simulink model "PMSM_Rs"  (R2024a)
settings: Solver=FixedStepDiscrete  StartTime=0.0  StopTime=0.5  FixedStep=1E-6  RelTol=1e-3
model workspace (MAT data in the model file):
  PWM_Frequency = Simulink.Parameter
  PWM_Frequency.Value = 30000
  PWM_Frequency.Complexity = 'real'
  PWM_Frequency.Dimensions = [1 1]
  PWM_Frequency.DataType = 'double'
  TimerPeriod = 0.1
values from neighbouring files (symbols this model uses):
  Flux = 0.01837    [Flux_Nonsensor_data_new.m]
undefined symbols (not defined in the file or in its folder): Down, Up
libraries: eePwmGenerator x11, slpidlib x3, spsDCVoltageSourceLib x2, spsPermanentMagnetSynchronousMachineLib x2, spsUniversalBridgeLib x2, sps_lib x1
settings Model: Creator=shish  LastModifiedBy=Administrator

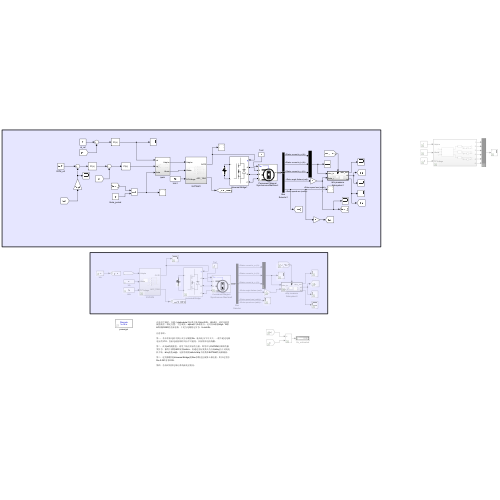
[thumbnail: Simulink's stored preview of the top-level diagram]
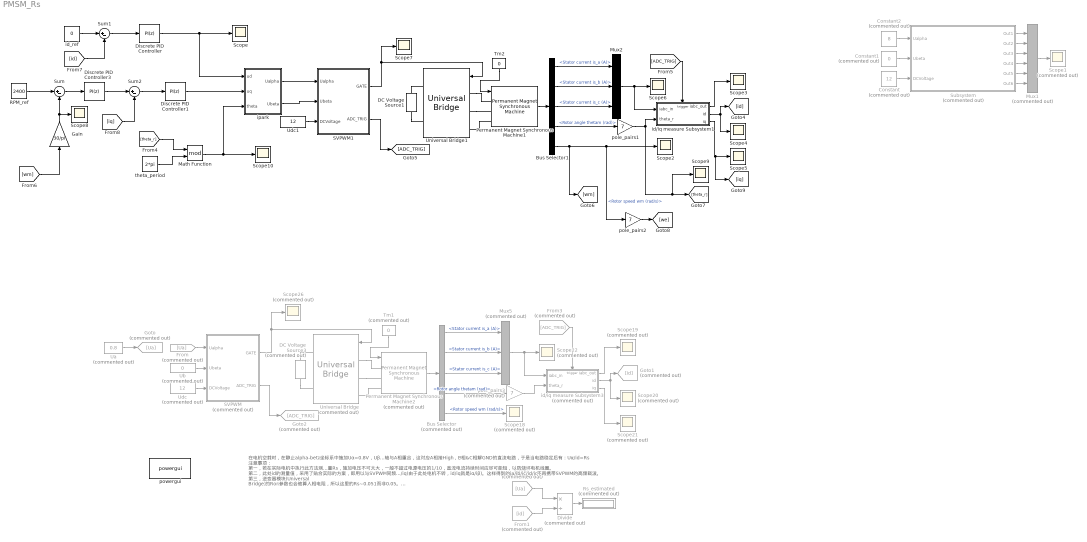
== system PMSM_Rs ==
  note: 在电机空载时，在静止alpha-beta坐标系中施加Uα=0.8V，Uβ=0V，此时电机将被强拖至一固定位置，不会旋转。alpha轴与A相重合，这对应A相接High，B相&C相解GND的直流电路，于是当电路稳定后有：Uα/id=Rs
      |
      | 注意事项：
      |
      | 第一，若在实际电机中执行此方法测量Rs，施加电压不可太大，一般不超过电源电压的1/10，直流电流持续时间应尽可能短，以防烧坏电机线圈。
      |
      | 第二，此处id的测量值，采用了贴合实际的方案，即用以与SVPWM同频率的触发信号，触发下桥臂ADC采样ia/ib/ic，再通过坐标变换人为合成id/iq(由于此处电机不转，id/iq就是iα/iβ)。这样得到的ia/ib/ic/id/iq不再携带SVPWM的高频载波。
      |
      | 第三，逆变器模块(Universal Bridge)的Ron参数也会被算入相电阻，所以这里的Rs~0.051而非0.05。
      |
      | 第四，仿真时间要足够让系统演化至稳态。
  Bus Selector : BusSelector  Commented=on  OutputSignals=Stator current is_a (A),Stator current is_b (A),Stator current is_c (A),Rotor angle thetam (rad),Rotor speed wm (rad/s)
  Bus Selector1 : BusSelector  OutputSignals=Stator current is_a (A),Stator current is_b (A),Stator current is_c (A),Rotor angle thetam (rad),Rotor speed wm (rad/s)
  Constant : Constant  Commented=on  Value=12
  Constant1 : Constant  Commented=on  Value=0
  Constant2 : Constant  Commented=on  Value=8
  DC Voltage Source1 : spsDCVoltageSourceLib/DC Voltage Source  Amplitude=12  Measurements=None
  DC Voltage Source3 : spsDCVoltageSourceLib/DC Voltage Source  Commented=on  Amplitude=12  Measurements=None
  Discrete PID Controller : slpidlib/PID Controller  Controller=PI  Form=Parallel  TimeDomain=Discrete-time  UseExternalTs=off  SampleTime=-1  IntegratorMethod=Forward Euler  FilterMethod=Forward Euler  ControllerParametersSource=internal  P=1000  I=5  UseKiTs=off  D=0  UseExternalDerivativeSource=off  N=100  UseFilter=on  TunerSelectOption=Transfer Function Based (PID Tuner App)  InitialConditionSource=internal  InitialConditionForIntegrator=0  InitialConditionForFilter=0  DifferentiatorICPrevScaledInput=0  ExternalReset=none  TrackingMode=off  Kt=1  LimitOutput=off  SatLimitsSource=internal  UpperSaturationLimit=inf  LowerSaturationLimit=-inf  LinearizeAsGain=off  AntiWindupMode=none  Kb=1  LimitIntegrator=off  UpperIntegratorSaturationLimit=inf  LowerIntegratorSaturationLimit=-inf  POutMin=[]  POutMax=[]  IOutMin=[]  IOutMax=[]  DOutMin=[]  DOutMax=[]  NOutMin=[]  NOutMax=[]  SumOutMin=[]  SumOutMax=[]  SaturationOutMin=[]  SaturationOutMax=[]  PParamMin=[]  PParamMax=[]  IParamMin=[]  IParamMax=[]  DParamMin=[]  DParamMax=[]  NParamMin=[]  NParamMax=[]  KbParamMin=[]  KbParamMax=[]  KtParamMin=[]  KtParamMax=[]  KbOutMin=[]  KbOutMax=[]  KtOutMin=[]  KtOutMax=[]  IntegratorOutMin=[]  IntegratorOutMax=[]  FilterOutMin=[]  FilterOutMax=[]  SumI1OutMin=[]  SumI1OutMax=[]  SumI2OutMin=[]  SumI2OutMax=[]  SumI3OutMin=[]  SumI3OutMax=[]  SumI4OutMin=[]  SumI4OutMax=[]  SumDOutMin=[]  SumDOutMax=[]  DifferentiatorOutMin=[]  DifferentiatorOutMax=[]  FilterDiffOutCoefMin=[]  FilterDiffOutCoefMax=[]  ReciprocalOutMin=[]  ReciprocalOutMax=[]  SumDenOutMin=[]  SumDenOutMax=[]  SumNumOutMin=[]  SumNumOutMax=[]  DivideOutMin=[]  DivideOutMax=[]  UdiffTsProdOutMin=[]  UdiffTsProdOutMax=[]  NTsProdOutMin=[]  NTsProdOutMax=[]  UintegralTsProdOutMin=[]  UintegralTsProdOutMax=[]  UngainTsProdOutMin=[]  UngainTsProdOutMax=[]  ClampingZeroOutDataTypeStr=Inherit: Inherit via back propagation  ClampingZeroOutMin=[]  ClampingZeroOutMax=[]  FilterDenConstantOutDataTypeStr=Inherit: Inherit via back propagation  FilterDenConstantOutMin=[]  FilterDenConstantOutMax=[]  PCopyOutDataTypeStr=Inherit: Inherit via back propagation  PCopyOutMin=[]  PCopyOutMax=[]  NCopyOutDataTypeStr=Inherit: Inherit via back propagation  NCopyOutMin=[]  NCopyOutMax=[]  IntegratorContinuousStateAttributes=''  IntegratorStateMustResolveToSignalObject=off  IntegratorRTWStateStorageClass=Auto  FilterContinuousStateAttributes=''  FilterStateMustResolveToSignalObject=off  FilterRTWStateStorageClass=Auto  ParallelPVariant=InternalParameters  IdealPVariant=Disabled  IVariant=InternalParameters  DVariant=Disabled  IntegratorVariant=Discrete  SatVariant=Disabled  AWVariant=Passthrough  PCopyVariant=Disabled  TRVariant=Disabled  FdbkBlocksVariant=Forward  IdealPFdbkVariant=Disabled  SatFdbkVariant=Disabled  DerivativeFilterVariant=Disabled  NVariant=Disabled  NCopyVariant=Disabled_SignalSpec  FilterICVariant=Disabled  IntegratorICVariant=InternalICs  ExternalResetVariant=Disabled  TRSumVariant=Passthrough  SumFdbkVariant=Disabled  SumVariant=Sum_PI  TsampFilterVariant=InternalTs  TsampNgainVariant=Passthrough  TsampIntegralVariant=Disabled_SignalSpec  ExternalSaturationOutDataTypeStr=Inherit: Same as second input  DerivativeSourceVariant=Disabled
      settings: LibrarySourceBlock=simulink/Discrete/Discrete PID Controller
  Discrete PID Controller1 : slpidlib/PID Controller  Controller=PI  Form=Parallel  TimeDomain=Discrete-time  UseExternalTs=off  SampleTime=-1  IntegratorMethod=Forward Euler  FilterMethod=Forward Euler  ControllerParametersSource=internal  P=1500  I=20  UseKiTs=off  D=0  UseExternalDerivativeSource=off  N=100  UseFilter=on  TunerSelectOption=Transfer Function Based (PID Tuner App)  InitialConditionSource=internal  InitialConditionForIntegrator=0  InitialConditionForFilter=0  DifferentiatorICPrevScaledInput=0  ExternalReset=none  TrackingMode=off  Kt=1  LimitOutput=off  SatLimitsSource=internal  UpperSaturationLimit=inf  LowerSaturationLimit=-inf  LinearizeAsGain=off  AntiWindupMode=none  Kb=1  LimitIntegrator=off  UpperIntegratorSaturationLimit=inf  LowerIntegratorSaturationLimit=-inf  POutMin=[]  POutMax=[]  IOutMin=[]  IOutMax=[]  DOutMin=[]  DOutMax=[]  NOutMin=[]  NOutMax=[]  SumOutMin=[]  SumOutMax=[]  SaturationOutMin=[]  SaturationOutMax=[]  PParamMin=[]  PParamMax=[]  IParamMin=[]  IParamMax=[]  DParamMin=[]  DParamMax=[]  NParamMin=[]  NParamMax=[]  KbParamMin=[]  KbParamMax=[]  KtParamMin=[]  KtParamMax=[]  KbOutMin=[]  KbOutMax=[]  KtOutMin=[]  KtOutMax=[]  IntegratorOutMin=[]  IntegratorOutMax=[]  FilterOutMin=[]  FilterOutMax=[]  SumI1OutMin=[]  SumI1OutMax=[]  SumI2OutMin=[]  SumI2OutMax=[]  SumI3OutMin=[]  SumI3OutMax=[]  SumI4OutMin=[]  SumI4OutMax=[]  SumDOutMin=[]  SumDOutMax=[]  DifferentiatorOutMin=[]  DifferentiatorOutMax=[]  FilterDiffOutCoefMin=[]  FilterDiffOutCoefMax=[]  ReciprocalOutMin=[]  ReciprocalOutMax=[]  SumDenOutMin=[]  SumDenOutMax=[]  SumNumOutMin=[]  SumNumOutMax=[]  DivideOutMin=[]  DivideOutMax=[]  UdiffTsProdOutMin=[]  UdiffTsProdOutMax=[]  NTsProdOutMin=[]  NTsProdOutMax=[]  UintegralTsProdOutMin=[]  UintegralTsProdOutMax=[]  UngainTsProdOutMin=[]  UngainTsProdOutMax=[]  ClampingZeroOutDataTypeStr=Inherit: Inherit via back propagation  ClampingZeroOutMin=[]  ClampingZeroOutMax=[]  FilterDenConstantOutDataTypeStr=Inherit: Inherit via back propagation  FilterDenConstantOutMin=[]  FilterDenConstantOutMax=[]  PCopyOutDataTypeStr=Inherit: Inherit via back propagation  PCopyOutMin=[]  PCopyOutMax=[]  NCopyOutDataTypeStr=Inherit: Inherit via back propagation  NCopyOutMin=[]  NCopyOutMax=[]  IntegratorContinuousStateAttributes=''  IntegratorStateMustResolveToSignalObject=off  IntegratorRTWStateStorageClass=Auto  FilterContinuousStateAttributes=''  FilterStateMustResolveToSignalObject=off  FilterRTWStateStorageClass=Auto  ParallelPVariant=InternalParameters  IdealPVariant=Disabled  IVariant=InternalParameters  DVariant=Disabled  IntegratorVariant=Discrete  SatVariant=Disabled  AWVariant=Passthrough  PCopyVariant=Disabled  TRVariant=Disabled  FdbkBlocksVariant=Forward  IdealPFdbkVariant=Disabled  SatFdbkVariant=Disabled  DerivativeFilterVariant=Disabled  NVariant=Disabled  NCopyVariant=Disabled_SignalSpec  FilterICVariant=Disabled  IntegratorICVariant=InternalICs  ExternalResetVariant=Disabled  TRSumVariant=Passthrough  SumFdbkVariant=Disabled  SumVariant=Sum_PI  TsampFilterVariant=InternalTs  TsampNgainVariant=Passthrough  TsampIntegralVariant=Disabled_SignalSpec  ExternalSaturationOutDataTypeStr=Inherit: Same as second input  DerivativeSourceVariant=Disabled
      settings: LibrarySourceBlock=simulink/Discrete/Discrete PID Controller
  Discrete PID Controller3 : slpidlib/PID Controller  Controller=PI  Form=Parallel  TimeDomain=Discrete-time  UseExternalTs=off  SampleTime=-1  IntegratorMethod=Forward Euler  FilterMethod=Forward Euler  ControllerParametersSource=internal  P=1500  I=10  UseKiTs=off  D=0  UseExternalDerivativeSource=off  N=100  UseFilter=on  TunerSelectOption=Transfer Function Based (PID Tuner App)  InitialConditionSource=internal  InitialConditionForIntegrator=0  InitialConditionForFilter=0  DifferentiatorICPrevScaledInput=0  ExternalReset=none  TrackingMode=off  Kt=1  LimitOutput=off  SatLimitsSource=internal  UpperSaturationLimit=inf  LowerSaturationLimit=-inf  LinearizeAsGain=off  AntiWindupMode=none  Kb=1  LimitIntegrator=off  UpperIntegratorSaturationLimit=inf  LowerIntegratorSaturationLimit=-inf  POutMin=[]  POutMax=[]  IOutMin=[]  IOutMax=[]  DOutMin=[]  DOutMax=[]  NOutMin=[]  NOutMax=[]  SumOutMin=[]  SumOutMax=[]  SaturationOutMin=[]  SaturationOutMax=[]  PParamMin=[]  PParamMax=[]  IParamMin=[]  IParamMax=[]  DParamMin=[]  DParamMax=[]  NParamMin=[]  NParamMax=[]  KbParamMin=[]  KbParamMax=[]  KtParamMin=[]  KtParamMax=[]  KbOutMin=[]  KbOutMax=[]  KtOutMin=[]  KtOutMax=[]  IntegratorOutMin=[]  IntegratorOutMax=[]  FilterOutMin=[]  FilterOutMax=[]  SumI1OutMin=[]  SumI1OutMax=[]  SumI2OutMin=[]  SumI2OutMax=[]  SumI3OutMin=[]  SumI3OutMax=[]  SumI4OutMin=[]  SumI4OutMax=[]  SumDOutMin=[]  SumDOutMax=[]  DifferentiatorOutMin=[]  DifferentiatorOutMax=[]  FilterDiffOutCoefMin=[]  FilterDiffOutCoefMax=[]  ReciprocalOutMin=[]  ReciprocalOutMax=[]  SumDenOutMin=[]  SumDenOutMax=[]  SumNumOutMin=[]  SumNumOutMax=[]  DivideOutMin=[]  DivideOutMax=[]  UdiffTsProdOutMin=[]  UdiffTsProdOutMax=[]  NTsProdOutMin=[]  NTsProdOutMax=[]  UintegralTsProdOutMin=[]  UintegralTsProdOutMax=[]  UngainTsProdOutMin=[]  UngainTsProdOutMax=[]  ClampingZeroOutDataTypeStr=Inherit: Inherit via back propagation  ClampingZeroOutMin=[]  ClampingZeroOutMax=[]  FilterDenConstantOutDataTypeStr=Inherit: Inherit via back propagation  FilterDenConstantOutMin=[]  FilterDenConstantOutMax=[]  PCopyOutDataTypeStr=Inherit: Inherit via back propagation  PCopyOutMin=[]  PCopyOutMax=[]  NCopyOutDataTypeStr=Inherit: Inherit via back propagation  NCopyOutMin=[]  NCopyOutMax=[]  IntegratorContinuousStateAttributes=''  IntegratorStateMustResolveToSignalObject=off  IntegratorRTWStateStorageClass=Auto  FilterContinuousStateAttributes=''  FilterStateMustResolveToSignalObject=off  FilterRTWStateStorageClass=Auto  ParallelPVariant=InternalParameters  IdealPVariant=Disabled  IVariant=InternalParameters  DVariant=Disabled  IntegratorVariant=Discrete  SatVariant=Disabled  AWVariant=Passthrough  PCopyVariant=Disabled  TRVariant=Disabled  FdbkBlocksVariant=Forward  IdealPFdbkVariant=Disabled  SatFdbkVariant=Disabled  DerivativeFilterVariant=Disabled  NVariant=Disabled  NCopyVariant=Disabled_SignalSpec  FilterICVariant=Disabled  IntegratorICVariant=InternalICs  ExternalResetVariant=Disabled  TRSumVariant=Passthrough  SumFdbkVariant=Disabled  SumVariant=Sum_PI  TsampFilterVariant=InternalTs  TsampNgainVariant=Passthrough  TsampIntegralVariant=Disabled_SignalSpec  ExternalSaturationOutDataTypeStr=Inherit: Same as second input  DerivativeSourceVariant=Disabled
      settings: LibrarySourceBlock=simulink/Discrete/Discrete PID Controller
  Divide : Product  Commented=on  Inputs=*/
  From : From  Commented=on  GotoTag=Ua
  From1 : From  Commented=on  GotoTag=id
  From2 : From  Commented=on  GotoTag=Ua
  From3 : From  Commented=on  GotoTag=ADC_TRIG
  Gain : Gain  Gain=30/pi
  Goto : Goto  Commented=on  GotoTag=Ua
  Goto1 : Goto  Commented=on  GotoTag=id
  Goto2 : Goto  Commented=on  GotoTag=ADC_TRIG
  Math Function : Math  Operator=mod
  Mux1 : Mux  Commented=on  Inputs=6
  Mux2 : Mux  Inputs=3
  Mux5 : Mux  Commented=on  Inputs=3
  Permanent Magnet Synchronous Machine1 : spsPermanentMagnetSynchronousMachineLib/Permanent Magnet Synchronous Machine  NbPhases=3  FluxDistribution=Sinusoidal  RotorType=Salient-pole  MechanicalLoad=Torque Tm  PresetModel=No  ShowDetailedParameters=on  MeasurementBus=off  Resistance=0.05  Inductance=8.5e-3  dqInductances=[1.8e-3,1.8e-3]  La=0.000395  MachineConstant=Flux linkage established by magnets (V.s)  Flux=0.00012  VoltageCst=0.15236  TorqueCst=0.00126  Flat=120  Mechanical=[0.000012 0.000005 7 0]  PolePairs=4  InitialConditions=[0,0, 0,0]  InitialConditions5ph=[0 0 0 0 0 0]  RefAngle=Aligned with phase A axis (original Park)  IterativeDiscreteModel=Trapezoidal non iterative  TsBlock=-1  TsPowergui=0
  Permanent Magnet Synchronous Machine2 : spsPermanentMagnetSynchronousMachineLib/Permanent Magnet Synchronous Machine  Commented=on  NbPhases=3  FluxDistribution=Sinusoidal  RotorType=Salient-pole  MechanicalLoad=Torque Tm  PresetModel=No  ShowDetailedParameters=on  MeasurementBus=off  Resistance=0.05  Inductance=8.5e-3  dqInductances=[1.8e-3,1.8e-3]  La=0.000395  MachineConstant=Flux linkage established by magnets (V.s)  Flux=0.00012  VoltageCst=0.15236  TorqueCst=0.00126  Flat=120  Mechanical=[0.000012 0.000005 7 0]  PolePairs=4  InitialConditions=[0,0, 0,0]  InitialConditions5ph=[0 0 0 0 0 0]  RefAngle=Aligned with phase A axis (original Park)  IterativeDiscreteModel=Trapezoidal non iterative  TsBlock=-1  TsPowergui=0
  RPM_ref : Constant  Value=2400
  Rs_estimated : Display  Commented=on
  SVPWM : Subsystem  Commented=on
  SVPWM1 : Subsystem
  Scope{,2..10} (10 alike) : Scope
  Scope{1,18..22,26} (7 alike) : Scope  Commented=on
  Subsystem : Subsystem  Commented=on
  Sum : Sum  Inputs=|+-
  Sum1 : Sum  Inputs=|+-
  Sum2 : Sum  Inputs=|+-
  Tm1 : Constant  Commented=on  Value=0
  Tm2 : Constant  Value=0
  Ua : Constant  Commented=on  Value=0.8
  Ub : Constant  Commented=on  Value=0
  Udc : Constant  Commented=on  Value=12
  Udc1 : Constant  Value=12
  Universal Bridge : spsUniversalBridgeLib/Universal Bridge  Commented=on  Arms=3  SnubberResistance=1e5  SnubberCapacitance=inf  Device=MOSFET / Diodes  Ron=1e-3  Lon=0  ForwardVoltages="[  0  0  ]"  ForwardVoltage=0  GTOparameters=[ 10e-6 , 20e-6 ]  IGBTparameters=[ 1e-6 , 2e-6 ]  Measurements=None  Measurements_2=None  converterType=Rectifier
  Universal Bridge1 : spsUniversalBridgeLib/Universal Bridge  Arms=3  SnubberResistance=1e5  SnubberCapacitance=inf  Device=MOSFET / Diodes  Ron=1e-3  Lon=0  ForwardVoltages="[  0  0  ]"  ForwardVoltage=0  GTOparameters=[ 10e-6 , 20e-6 ]  IGBTparameters=[ 1e-6 , 2e-6 ]  Measurements=None  Measurements_2=None  converterType=Rectifier
  id/iq measure Subsystem1 : Subsystem  TreatAsAtomicUnit=on
  id/iq measure Subsystem3 : Subsystem  Commented=on  TreatAsAtomicUnit=on
  id_ref : Constant  Value=0
  ipark : Subsystem
  pole_pairs1 : Gain  Gain=7
  pole_pairs2 : Gain  Gain=7
  pole_pairs3 : Gain  Commented=on  Gain=7
  powergui : sps_lib/powergui  Priority=1  SimulationMode=Discrete  SampleTime=1e-6  frequency=60  Iterations=50  frequencyindice=0  Pbase=100e6  ErrMax=1e-4  UnitsV=kV  UnitsW=MW  buscounter=0  FunctionMessages=off  echomessages=off  EnableUseOfTLC=off  CurrentSourceSwitches=off  DisableSnubberDevices=off  DisableRonSwitches=off  DisableVfSwitches=off  DisplayEquations=off  AutomaticDiscreteSolvers=off  SolverType=Tustin/Backward Euler (TBE)  Interpol=off  ExternalGateDelay=off  methode=off  Ts=100  x0status=blocks  SPID=on  SwTol=0  HookPort=off  NonlinearTolerance=1e-4  nMaxIteration=100  ContinueOnMaxIteration=off  RestoreLinks=warning  ResistiveCurrentMeasurement=off  Frange=[0:2:500]  Ylog=off  Xlog=on  ShowGrid=off  save=off  variable=ZData  structure=0  ZoomFFT=off  StartTime=0.0  cycles=1  DisplayStyle=1  fundamental=60  FreqAxis=off  MaxFrequency=1000  frequencyindicesteady=1  RmsSteady=1  display=off
  theta_period : Constant  Value=2*pi
  wires:
  Subsystem/1(Out1) -> Mux1/1
  Subsystem/2(Out2) -> Mux1/2
  Subsystem/3(Out3) -> Mux1/3
  Subsystem/4(Out4) -> Mux1/4
  Subsystem/5(Out5) -> Mux1/5
  Subsystem/6(Out6) -> Mux1/6
  Mux1/1 -> Scope1/1
  Constant/1 -> Subsystem/3(DCVoltage)
  Constant2/1 -> Subsystem/1(Ualpha)
  Constant1/1 -> Subsystem/2(Ubeta)
  Bus Selector/5 -> Scope18/1  "<Rotor speed wm (rad/s)>"
  Bus Selector/3 -> Mux5/3  "<Stator current is_c (A)>"
  Permanent Magnet Synchronous Machine2/1 -> Bus Selector/1
  Bus Selector/4 -> pole_pairs3/1  "<Rotor angle thetam (rad)>"
  Udc/1 -> SVPWM/3(DCVoltage)
  id/iq measure Subsystem3/1(iabc_out) -> Scope19/1
  Bus Selector/2 -> Mux5/2  "<Stator current is_b (A)>"
  Mux5/1 -> Scope22/1, id/iq measure Subsystem3/1(iabc_in)
  Tm1/1 -> Permanent Magnet Synchronous Machine2/1
  SVPWM/1(GATE) -> Universal Bridge/1, Scope26/1
  Bus Selector/1 -> Mux5/1  "<Stator current is_a (A)>"
  pole_pairs3/1 -> id/iq measure Subsystem3/2(theta_r)
  id/iq measure Subsystem3/2(id) -> Goto1/1, Scope20/1
  id/iq measure Subsystem3/3(iq) -> Scope21/1
  Ub/1 -> SVPWM/2(Ubeta)
  From/1 -> SVPWM/1(Ualpha)
  Ua/1 -> Goto/1
  From2/1 -> Divide/1
  From1/1 -> Divide/2
  Divide/1 -> Rs_estimated/1
  SVPWM/2(ADC_TRIG) -> Goto2/1
  From3/1 -> id/iq measure Subsystem3/Trigger
  [ADC_TRIG] -> id/iq measure Subsystem1/Trigger
  Tm2/1 -> Permanent Magnet Synchronous Machine1/1
  Bus Selector1/2 -> Mux2/2  "<Stator current is_b (A)>"
  Bus Selector1/1 -> Mux2/1  "<Stator current is_a (A)>"
  Bus Selector1/3 -> Mux2/3  "<Stator current is_c (A)>"
  id/iq measure Subsystem1/3(iq) -> [iq], Scope5/1
  SVPWM1/2(ADC_TRIG) -> [ADC_TRIG]
  id/iq measure Subsystem1/2(id) -> [id], Scope4/1
  Mux2/1 -> Scope6/1, id/iq measure Subsystem1/1(iabc_in)
  ipark/1(Ualpha) -> SVPWM1/1(Ualpha)
  id/iq measure Subsystem1/1(iabc_out) -> Scope3/1
  Permanent Magnet Synchronous Machine1/1 -> Bus Selector1/1
  Bus Selector1/5 -> pole_pairs2/1, Scope2/1, [wm]  "<Rotor speed wm (rad/s)>"
  Bus Selector1/4 -> pole_pairs1/1  "<Rotor angle thetam (rad)>"
  Udc1/1 -> SVPWM1/3(DCVoltage)
  pole_pairs1/1 -> Scope9/1, [theta_r], id/iq measure Subsystem1/2(theta_r)
  SVPWM1/1(GATE) -> Universal Bridge1/1, Scope7/1
  pole_pairs2/1 -> [we]
  [wm] -> Gain/1
  Sum/1 -> Discrete PID Controller3/1
  [id] -> Sum1/2
  Sum1/1 -> Discrete PID Controller/1
  [iq] -> Sum2/2
  id_ref/1 -> Sum1/1
  ipark/2(Ubeta) -> SVPWM1/2(Ubeta)
  Discrete PID Controller/1 -> ipark/1(ud), Scope/1
  Gain/1 -> Sum/2, Scope8/1
  RPM_ref/1 -> Sum/1
  Discrete PID Controller3/1 -> Sum2/1
  Sum2/1 -> Discrete PID Controller1/1
  Discrete PID Controller1/1 -> ipark/2(uq)
  [theta_r] -> Math Function/1
  theta_period/1 -> Math Function/2
  Math Function/1 -> Scope10/1, ipark/3(theta)
  connections:
  Universal Bridge/LConn2 -- Permanent Magnet Synchronous Machine2/LConn2
  Universal Bridge/LConn1 -- Permanent Magnet Synchronous Machine2/LConn1
  DC Voltage Source3/RConn1 -- Universal Bridge/RConn1
  Universal Bridge/LConn3 -- Permanent Magnet Synchronous Machine2/LConn3
  DC Voltage Source3/LConn1 -- Universal Bridge/RConn2
  DC Voltage Source1/LConn1 -- Universal Bridge1/RConn2
  Universal Bridge1/LConn1 -- Permanent Magnet Synchronous Machine1/LConn1
  Universal Bridge1/LConn3 -- Permanent Magnet Synchronous Machine1/LConn3
  DC Voltage Source1/RConn1 -- Universal Bridge1/RConn1
  Universal Bridge1/LConn2 -- Permanent Magnet Synchronous Machine1/LConn2

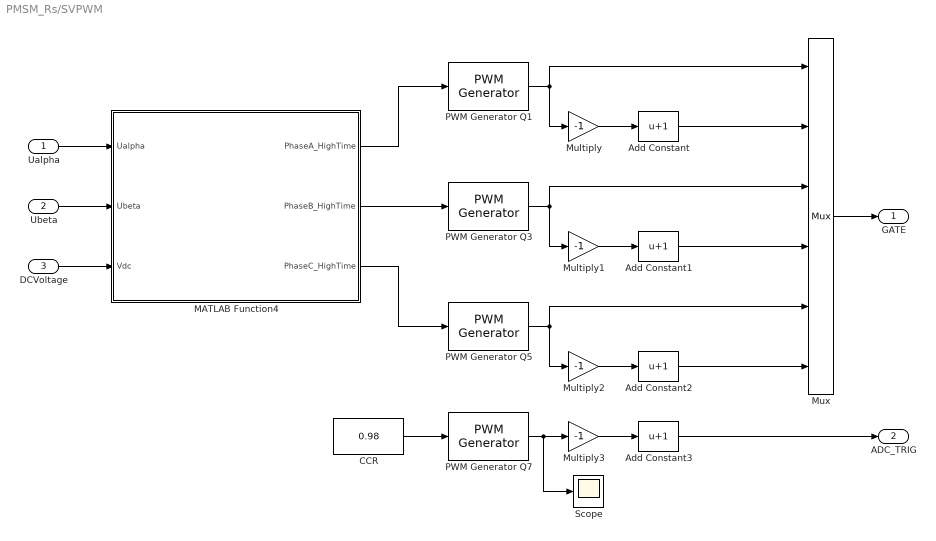
== system PMSM_Rs/SVPWM ==
  Ualpha : Inport
  Ubeta : Inport  Port=2
  DCVoltage : Inport  Port=3
  Add Constant{,1..3} (4 alike) : Bias  Bias=1  SaturateOnIntegerOverflow=off
  CCR : Constant  Value=0.98
  MATLAB Function4 : MATLAB Function  TreatAsAtomicUnit=on
  Multiply{,1..3} (4 alike) : Gain  Gain=-1
  Mux : Mux  Inputs=6
  PWM Generator Q{1,3,5,7} (4 alike) : eePwmGenerator/PWM Generator  CarrCount=Up-Down  Tper=1.0/PWM_Frequency  Tdelay=0  Ts=1E-6
  Scope : Scope
  GATE : Outport
  ADC_TRIG : Outport  Port=2
  wires:
  PWM Generator Q5/1 -> Mux/5, Multiply2/1
  PWM Generator Q1/1 -> Multiply/1, Mux/1
  Add Constant1/1 -> Mux/4
  Ubeta/1 -> MATLAB Function4/2(Ubeta)
  DCVoltage/1 -> MATLAB Function4/3(Vdc)
  MATLAB Function4/3(PhaseC_HighTime) -> PWM Generator Q5/1
  Multiply/1 -> Add Constant/1
  Multiply2/1 -> Add Constant2/1
  Add Constant/1 -> Mux/2
  MATLAB Function4/2(PhaseB_HighTime) -> PWM Generator Q3/1
  Add Constant2/1 -> Mux/6
  Multiply1/1 -> Add Constant1/1
  MATLAB Function4/1(PhaseA_HighTime) -> PWM Generator Q1/1
  Ualpha/1 -> MATLAB Function4/1(Ualpha)
  PWM Generator Q3/1 -> Mux/3, Multiply1/1
  PWM Generator Q7/1 -> Scope/1, Multiply3/1
  CCR/1 -> PWM Generator Q7/1
  Add Constant3/1 -> ADC_TRIG/1
  Multiply3/1 -> Add Constant3/1
  Mux/1 -> GATE/1

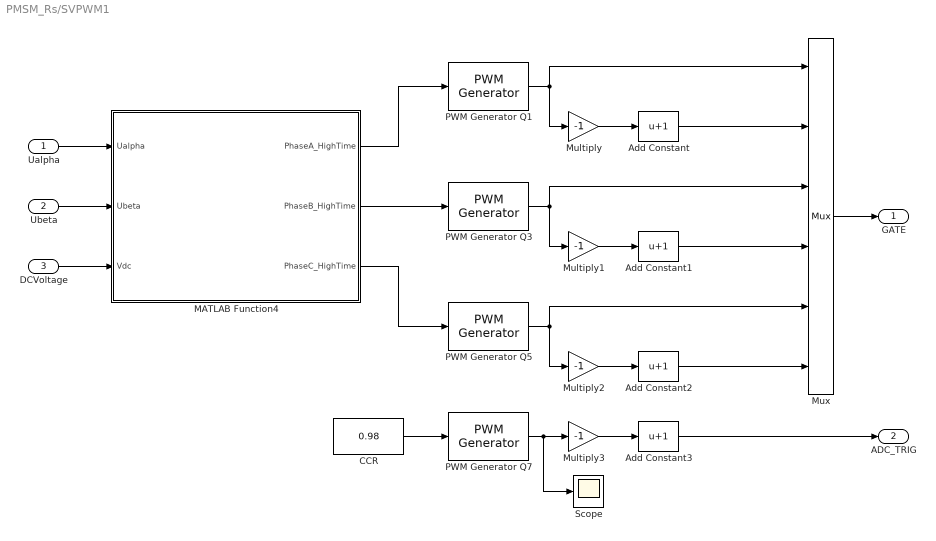
== system PMSM_Rs/SVPWM1 ==
  Ualpha : Inport
  Ubeta : Inport  Port=2
  DCVoltage : Inport  Port=3
  Add Constant{,1..3} (4 alike) : Bias  Bias=1  SaturateOnIntegerOverflow=off
  CCR : Constant  Value=0.98
  MATLAB Function4 : MATLAB Function  TreatAsAtomicUnit=on
  Multiply{,1..3} (4 alike) : Gain  Gain=-1
  Mux : Mux  Inputs=6
  PWM Generator Q{1,3,5,7} (4 alike) : eePwmGenerator/PWM Generator  CarrCount=Up-Down  Tper=1.0/PWM_Frequency  Tdelay=0  Ts=1E-6
  Scope : Scope
  GATE : Outport
  ADC_TRIG : Outport  Port=2
  wires:
  PWM Generator Q5/1 -> Mux/5, Multiply2/1
  PWM Generator Q1/1 -> Multiply/1, Mux/1
  Add Constant1/1 -> Mux/4
  Ubeta/1 -> MATLAB Function4/2(Ubeta)
  DCVoltage/1 -> MATLAB Function4/3(Vdc)
  MATLAB Function4/3(PhaseC_HighTime) -> PWM Generator Q5/1
  Multiply/1 -> Add Constant/1
  Multiply2/1 -> Add Constant2/1
  Add Constant/1 -> Mux/2
  MATLAB Function4/2(PhaseB_HighTime) -> PWM Generator Q3/1
  Add Constant2/1 -> Mux/6
  Multiply1/1 -> Add Constant1/1
  MATLAB Function4/1(PhaseA_HighTime) -> PWM Generator Q1/1
  Ualpha/1 -> MATLAB Function4/1(Ualpha)
  PWM Generator Q3/1 -> Mux/3, Multiply1/1
  PWM Generator Q7/1 -> Scope/1, Multiply3/1
  CCR/1 -> PWM Generator Q7/1
  Add Constant3/1 -> ADC_TRIG/1
  Multiply3/1 -> Add Constant3/1
  Mux/1 -> GATE/1

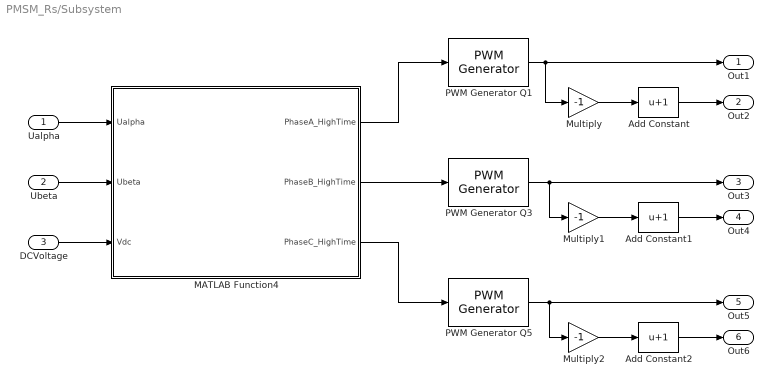
== system PMSM_Rs/Subsystem ==
  Ualpha : Inport
  Ubeta : Inport  Port=2
  DCVoltage : Inport  Port=3
  Add Constant : Bias  Bias=1  SaturateOnIntegerOverflow=off
  Add Constant1 : Bias  Bias=1  SaturateOnIntegerOverflow=off
  Add Constant2 : Bias  Bias=1  SaturateOnIntegerOverflow=off
  MATLAB Function4 : MATLAB Function  TreatAsAtomicUnit=on
  Multiply : Gain  Gain=-1
  Multiply1 : Gain  Gain=-1
  Multiply2 : Gain  Gain=-1
  PWM Generator Q1 : eePwmGenerator/PWM Generator  CarrCount=Up-Down  Tper=0.1  Tdelay=0  Ts=1E-5
  PWM Generator Q3 : eePwmGenerator/PWM Generator  CarrCount=Up-Down  Tper=0.1  Tdelay=0  Ts=1E-5
  PWM Generator Q5 : eePwmGenerator/PWM Generator  CarrCount=Up-Down  Tper=0.1  Tdelay=0  Ts=1E-5
  Out1 : Outport
  Out2 : Outport  Port=2
  Out3 : Outport  Port=3
  Out4 : Outport  Port=4
  Out5 : Outport  Port=5
  Out6 : Outport  Port=6
  wires:
  PWM Generator Q5/1 -> Out5/1, Multiply2/1
  PWM Generator Q1/1 -> Out1/1, Multiply/1
  Add Constant1/1 -> Out4/1
  Ubeta/1 -> MATLAB Function4/2(Ubeta)
  DCVoltage/1 -> MATLAB Function4/3(Vdc)
  MATLAB Function4/3(PhaseC_HighTime) -> PWM Generator Q5/1
  Multiply/1 -> Add Constant/1
  Multiply2/1 -> Add Constant2/1
  Add Constant/1 -> Out2/1
  MATLAB Function4/2(PhaseB_HighTime) -> PWM Generator Q3/1
  Add Constant2/1 -> Out6/1
  Multiply1/1 -> Add Constant1/1
  MATLAB Function4/1(PhaseA_HighTime) -> PWM Generator Q1/1
  Ualpha/1 -> MATLAB Function4/1(Ualpha)
  PWM Generator Q3/1 -> Out3/1, Multiply1/1

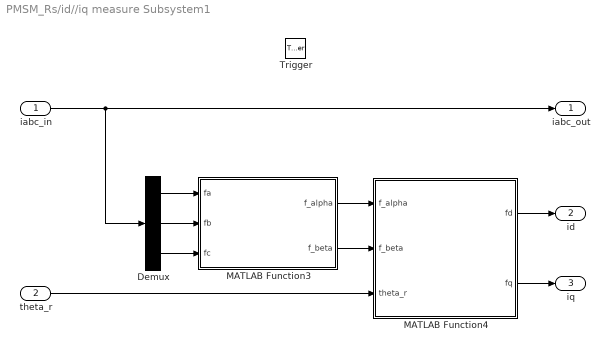
== system PMSM_Rs/id//iq measure Subsystem1 ==
  iabc_in : Inport
  theta_r : Inport  Port=2
  Trigger : TriggerPort  VariantControl=(inherit)
  Demux : Demux  Outputs=3
  MATLAB Function3 : MATLAB Function  TreatAsAtomicUnit=on
  MATLAB Function4 : MATLAB Function  TreatAsAtomicUnit=on
  iabc_out : Outport
  id : Outport  Port=2
  iq : Outport  Port=3
  wires:
  iabc_in/1 -> Demux/1, iabc_out/1
  Demux/3 -> MATLAB Function3/3(fc)
  Demux/2 -> MATLAB Function3/2(fb)
  Demux/1 -> MATLAB Function3/1(fa)
  MATLAB Function3/1(f_alpha) -> MATLAB Function4/1(f_alpha)
  MATLAB Function3/2(f_beta) -> MATLAB Function4/2(f_beta)
  theta_r/1 -> MATLAB Function4/3(theta_r)
  MATLAB Function4/1(fd) -> id/1
  MATLAB Function4/2(fq) -> iq/1

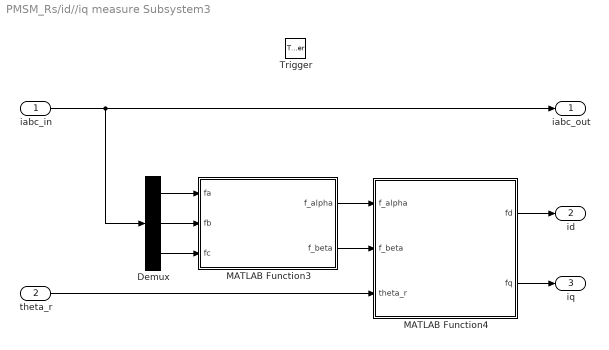
== system PMSM_Rs/id//iq measure Subsystem3 ==
  iabc_in : Inport
  theta_r : Inport  Port=2
  Trigger : TriggerPort  VariantControl=(inherit)
  Demux : Demux  Outputs=3
  MATLAB Function3 : MATLAB Function  TreatAsAtomicUnit=on
  MATLAB Function4 : MATLAB Function  TreatAsAtomicUnit=on
  iabc_out : Outport
  id : Outport  Port=2
  iq : Outport  Port=3
  wires:
  iabc_in/1 -> Demux/1, iabc_out/1
  Demux/3 -> MATLAB Function3/3(fc)
  Demux/2 -> MATLAB Function3/2(fb)
  Demux/1 -> MATLAB Function3/1(fa)
  MATLAB Function3/1(f_alpha) -> MATLAB Function4/1(f_alpha)
  MATLAB Function3/2(f_beta) -> MATLAB Function4/2(f_beta)
  theta_r/1 -> MATLAB Function4/3(theta_r)
  MATLAB Function4/1(fd) -> id/1
  MATLAB Function4/2(fq) -> iq/1

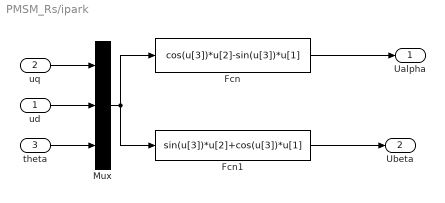
== system PMSM_Rs/ipark ==
  ud : Inport
  uq : Inport  Port=2
  theta : Inport  Port=3
  Fcn : Fcn  Expr=cos(u[3])*u[2]-sin(u[3])*u[1]
  Fcn1 : Fcn  Expr=sin(u[3])*u[2]+cos(u[3])*u[1]
  Mux : Mux  Inputs=3
  Ualpha : Outport
  Ubeta : Outport  Port=2
  wires:
  Mux/1 -> Fcn/1, Fcn1/1
  ud/1 -> Mux/2
  theta/1 -> Mux/3
  uq/1 -> Mux/1
  Fcn1/1 -> Ubeta/1
  Fcn/1 -> Ualpha/1

== matlab function PMSM_Rs/SVPWM1/MATLAB Function4 ==
  data: Ualpha input; PhaseA_HighTime output; Ubeta input; Vdc input; PhaseB_HighTime output; PhaseC_HighTime output
function [PhaseA_HighTime,PhaseB_HighTime,PhaseC_HighTime] = SVPWM_calculate(Ualpha,Ubeta,Vdc)

% unit:V %

%step 1,which sector?%
if Ualpha >= 0
    %sector=1,2,5,6%
    if Ubeta >= 0
        %sector=1,2%
        if Ubeta > sqrt(3)*Ualpha
            sector=2;
        else
            sector=1;
        end
    else
        %sector=5,6%
        if -Ubeta > sqrt(3)*Ualpha
            sector=5;
        else
            sector=6;
        end
    end
else
    %sector=2,3,4,5%
    if Ubeta >= 0
        %sector=2,3%
        if Ubeta > -sqrt(3)*Ualpha
            sector=2;
        else
            sector=3;
        end
    else
        %sector=4,5%
        if -Ubeta > -sqrt(3)*Ualpha
            sector=5;
        else
            sector=4;
        end
    end
end

%step 2,vector decompose%
v1 = (2*Vdc/3)*[ 1,0];
v2 = (2*Vdc/3)*[ 0.5, 0.5*sqrt(3)];
v3 = (2*Vdc/3)*[-0.5, 0.5*sqrt(3)];
v4 = (2*Vdc/3)*[-1,0];
v5 = (2*Vdc/3)*[-0.5,-0.5*sqrt(3)];
v6 = (2*Vdc/3)*[ 0.5,-0.5*sqrt(3)];

if sector == 1
    vm=v1;vn=v2;
elseif sector == 2
    vm=v2;vn=v3;
elseif sector == 3
    vm=v3;vn=v4;
elseif sector == 4
    vm=v4;vn=v5;
elseif sector == 5
    vm=v5;vn=v6;
else
    vm=v6;vn=v1;
end

cm = (Ualpha*vn(2) - Ubeta*vn(1))/(vm(1)*vn(2) - vm(2)*vn(1));

if abs(vn(1))>1e-7
    cn = (Ualpha-cm*vm(1))/vn(1);
else
    cn = (Ubeta-cm*vm(2))/vn(2);
end
c_summ = cm+cn;
% if c_summ > 1
%     cm = cm/c_summ;
%     cn = cn/c_summ;
% end
if c_summ > 0.95
    cm = 0.95*cm/c_summ;
    cn = 0.95*cn/c_summ;
end

c0 = (1-cm-cn);
c0 = 0.5*c0;
c7 = c0;

%step 3,duty cycle%
if sector == 1
    %v1:100  v2:110%
    PhaseA_HighTime = cm+cn+c7;
    PhaseB_HighTime = cn+c7;
    PhaseC_HighTime = c7;
elseif sector == 2
    %v2:110  v3:010%
    PhaseA_HighTime = cm+c7;
    PhaseB_HighTime = cm+cn+c7;
    PhaseC_HighTime = c7;
elseif sector == 3
    %v3:010  v4:011%
    PhaseA_HighTime = c7;
    PhaseB_HighTime = cm+cn+c7;
    PhaseC_HighTime = cn+c7;
elseif sector == 4
    %v4:011  v5:001%
    PhaseA_HighTime = c7;
    PhaseB_HighTime = cm+c7;
    PhaseC_HighTime = cm+cn+c7;
elseif sector == 5
    %v5:001  v6:101%
    PhaseA_HighTime = cn+c7;
    PhaseB_HighTime = c7;
    PhaseC_HighTime = cm+cn+c7;
else
    %v6:101  v1:100%
    PhaseA_HighTime = cm+cn+c7;
    PhaseB_HighTime = c7;
    PhaseC_HighTime = cm+c7;
end

== matlab function PMSM_Rs/id//iq measure Subsystem1/MATLAB Function3 ==
  data: fa input; f_alpha output; fb input; fc input; f_beta output
function [f_alpha,f_beta]= ABC_to_AlphaBeta(fa,fb,fc)
f_alpha = (2/3)*(fa-0.5*(fb+fc));
f_beta = (2/3)*(0.5*sqrt(3)*(fb-fc));

== matlab function PMSM_Rs/id//iq measure Subsystem1/MATLAB Function4 ==
  data: f_alpha input; fd output; f_beta input; fq output; theta_r input
function [fd,fq]= AlphaBeta_to_dq(f_alpha,f_beta,theta_r)

c = cos(theta_r);
s = sin(theta_r);
fd =  c*f_alpha + s*f_beta;
fq = -s*f_alpha + c*f_beta;

== matlab function PMSM_Rs/Subsystem/MATLAB Function4 ==
  data: Ualpha input; PhaseA_HighTime output; Ubeta input; Vdc input; PhaseB_HighTime output; PhaseC_HighTime output
function [PhaseA_HighTime,PhaseB_HighTime,PhaseC_HighTime] = SVPWM_calculate(Ualpha,Ubeta,Vdc)

% unit:V %

%step 1,which sector?%
if Ualpha >= 0
    %sector=1,2,5,6%
    if Ubeta >= 0
        %sector=1,2%
        if Ubeta > sqrt(3)*Ualpha
            sector=2;
        else
            sector=1;
        end
    else
        %sector=5,6%
        if -Ubeta > sqrt(3)*Ualpha
            sector=5;
        else
            sector=6;
        end
    end
else
    %sector=2,3,4,5%
    if Ubeta >= 0
        %sector=2,3%
        if Ubeta > -sqrt(3)*Ualpha
            sector=2;
        else
            sector=3;
        end
    else
        %sector=4,5%
        if -Ubeta > -sqrt(3)*Ualpha
            sector=5;
        else
            sector=4;
        end
    end
end

%step 2,vector decompose%
v1 = Vdc*[ 1,0];
v2 = Vdc*[ 0.5, 0.5*sqrt(3)];
v3 = Vdc*[-0.5, 0.5*sqrt(3)];
v4 = Vdc*[-1,0];
v5 = Vdc*[-0.5,-0.5*sqrt(3)];
v6 = Vdc*[ 0.5,-0.5*sqrt(3)];

if sector == 1
    vm=v1;vn=v2;
elseif sector == 2
    vm=v2;vn=v3;
elseif sector == 3
    vm=v3;vn=v4;
elseif sector == 4
    vm=v4;vn=v5;
elseif sector == 5
    vm=v5;vn=v6;
else
    vm=v6;vn=v1;
end

cm = (Ualpha*vn(2) - Ubeta*vn(1))/(vm(1)*vn(2) - vm(2)*vn(1));

if abs(vn(1))>1e-7
    cn = (Ualpha-cm*vm(1))/vn(1);
else
    cn = (Ubeta-cm*vm(2))/vn(2);
end
c_summ = cm+cn;
if c_summ > 1
    cm = cm/c_summ;
    cn = cn/c_summ;
end
c0 = (1-cm-cn);
c0 = 0.5*c0;
c7 = c0;

%step 3,duty cycle%
if sector == 1
    %v1:100  v2:110%
    PhaseA_HighTime = cm+cn+c7;
    PhaseB_HighTime = cn+c7;
    PhaseC_HighTime = c7;
elseif sector == 2
    %v2:110  v3:010%
    PhaseA_HighTime = cm+c7;
    PhaseB_HighTime = cm+cn+c7;
    PhaseC_HighTime = c7;
elseif sector == 3
    %v3:010  v4:011%
    PhaseA_HighTime = c7;
    PhaseB_HighTime = cm+cn+c7;
    PhaseC_HighTime = cn+c7;
elseif sector == 4
    %v4:011  v5:001%
    PhaseA_HighTime = c7;
    PhaseB_HighTime = cm+c7;
    PhaseC_HighTime = cm+cn+c7;
elseif sector == 5
    %v5:001  v6:101%
    PhaseA_HighTime = cn+c7;
    PhaseB_HighTime = c7;
    PhaseC_HighTime = cm+cn+c7;
else
    %v6:101  v1:100%
    PhaseA_HighTime = cm+cn+c7;
    PhaseB_HighTime = c7;
    PhaseC_HighTime = cm+c7;
end

== matlab function PMSM_Rs/SVPWM/MATLAB Function4 ==
  data: Ualpha input; PhaseA_HighTime output; Ubeta input; Vdc input; PhaseB_HighTime output; PhaseC_HighTime output
function [PhaseA_HighTime,PhaseB_HighTime,PhaseC_HighTime] = SVPWM_calculate(Ualpha,Ubeta,Vdc)

% unit:V %

%step 1,which sector?%
if Ualpha >= 0
    %sector=1,2,5,6%
    if Ubeta >= 0
        %sector=1,2%
        if Ubeta > sqrt(3)*Ualpha
            sector=2;
        else
            sector=1;
        end
    else
        %sector=5,6%
        if -Ubeta > sqrt(3)*Ualpha
            sector=5;
        else
            sector=6;
        end
    end
else
    %sector=2,3,4,5%
    if Ubeta >= 0
        %sector=2,3%
        if Ubeta > -sqrt(3)*Ualpha
            sector=2;
        else
            sector=3;
        end
    else
        %sector=4,5%
        if -Ubeta > -sqrt(3)*Ualpha
            sector=5;
        else
            sector=4;
        end
    end
end

%step 2,vector decompose%
v1 = (2*Vdc/3)*[ 1,0];
v2 = (2*Vdc/3)*[ 0.5, 0.5*sqrt(3)];
v3 = (2*Vdc/3)*[-0.5, 0.5*sqrt(3)];
v4 = (2*Vdc/3)*[-1,0];
v5 = (2*Vdc/3)*[-0.5,-0.5*sqrt(3)];
v6 = (2*Vdc/3)*[ 0.5,-0.5*sqrt(3)];

if sector == 1
    vm=v1;vn=v2;
elseif sector == 2
    vm=v2;vn=v3;
elseif sector == 3
    vm=v3;vn=v4;
elseif sector == 4
    vm=v4;vn=v5;
elseif sector == 5
    vm=v5;vn=v6;
else
    vm=v6;vn=v1;
end

cm = (Ualpha*vn(2) - Ubeta*vn(1))/(vm(1)*vn(2) - vm(2)*vn(1));

if abs(vn(1))>1e-7
    cn = (Ualpha-cm*vm(1))/vn(1);
else
    cn = (Ubeta-cm*vm(2))/vn(2);
end
c_summ = cm+cn;
% if c_summ > 1
%     cm = cm/c_summ;
%     cn = cn/c_summ;
% end
if c_summ > 0.95
    cm = 0.95*cm/c_summ;
    cn = 0.95*cn/c_summ;
end

c0 = (1-cm-cn);
c0 = 0.5*c0;
c7 = c0;

%step 3,duty cycle%
if sector == 1
    %v1:100  v2:110%
    PhaseA_HighTime = cm+cn+c7;
    PhaseB_HighTime = cn+c7;
    PhaseC_HighTime = c7;
elseif sector == 2
    %v2:110  v3:010%
    PhaseA_HighTime = cm+c7;
    PhaseB_HighTime = cm+cn+c7;
    PhaseC_HighTime = c7;
elseif sector == 3
    %v3:010  v4:011%
    PhaseA_HighTime = c7;
    PhaseB_HighTime = cm+cn+c7;
    PhaseC_HighTime = cn+c7;
elseif sector == 4
    %v4:011  v5:001%
    PhaseA_HighTime = c7;
    PhaseB_HighTime = cm+c7;
    PhaseC_HighTime = cm+cn+c7;
elseif sector == 5
    %v5:001  v6:101%
    PhaseA_HighTime = cn+c7;
    PhaseB_HighTime = c7;
    PhaseC_HighTime = cm+cn+c7;
else
    %v6:101  v1:100%
    PhaseA_HighTime = cm+cn+c7;
    PhaseB_HighTime = c7;
    PhaseC_HighTime = cm+c7;
end

== matlab function PMSM_Rs/id//iq measure Subsystem3/MATLAB Function3 ==
  data: fa input; f_alpha output; fb input; fc input; f_beta output
function [f_alpha,f_beta]= ABC_to_AlphaBeta(fa,fb,fc)
f_alpha = (2/3)*(fa-0.5*(fb+fc));
f_beta = (2/3)*(0.5*sqrt(3)*(fb-fc));

== matlab function PMSM_Rs/id//iq measure Subsystem3/MATLAB Function4 ==
  data: f_alpha input; fd output; f_beta input; fq output; theta_r input
function [fd,fq]= AlphaBeta_to_dq(f_alpha,f_beta,theta_r)

c = cos(theta_r);
s = sin(theta_r);
fd =  c*f_alpha + s*f_beta;
fq = -s*f_alpha + c*f_beta;
